simulink model "discrete_kalman_filter"  (R2015b)
settings: Solver=VariableStepAuto  StartTime=0.0  StopTime=10.0  RelTol=1e-3
undefined symbols (not defined in the file or in its folder): KF_A, KF_B, KF_C, KF_D, KF_h, KF_P0, KF_Q, KF_R, KF_x0
settings Model: Creator=mgreiff  LastModifiedBy=mgreiff

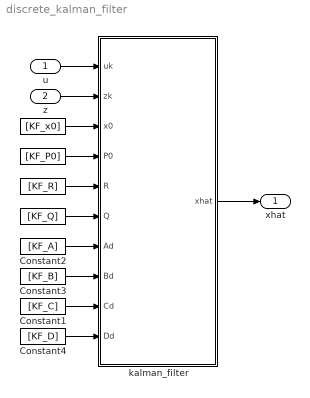
== system discrete_kalman_filter ==
  u : Inport  PortDimensions=4
  z : Inport  Port=2  PortDimensions=9
  " " : Constant  Value=[KF_P0]
  "  " : Constant  Value=[KF_R]
  "   " : Constant  Value=[KF_Q]
  "          " : Constant  Value=[KF_x0]
  Constant1 : Constant  Value=[KF_C]
  Constant2 : Constant  Value=[KF_A]
  Constant3 : Constant  Value=[KF_B]
  Constant4 : Constant  Value=[KF_D]
  kalman_filter : MATLAB Function  TreatAsAtomicUnit=on  SystemSampleTime=KF_h
  xhat : Outport  PortDimensions=12
  wires:
  u/1 -> kalman_filter/1(uk)
  z/1 -> kalman_filter/2(zk)
  " "/1 -> kalman_filter/4(P0)
  "  "/1 -> kalman_filter/5(R)
  "   "/1 -> kalman_filter/6(Q)
  kalman_filter/1(xhat) -> xhat/1
  Constant1/1 -> kalman_filter/9(Cd)
  "          "/1 -> kalman_filter/3(x0)
  Constant4/1 -> kalman_filter/10(Dd)
  Constant3/1 -> kalman_filter/8(Bd)
  Constant2/1 -> kalman_filter/7(Ad)

== matlab function discrete_kalman_filter/kalman_filter ==
  data: uk input; zk input; xhat output; x0 input; P0 input; R input; Q input; Ad input; Bd input; Cd input; Dd input
function xhat  = fcn(uk, zk, x0, P0, R, Q, Ad, Bd, Cd, Dd)
%#codegen
% xkm1  = [x,             uk = [omega_1,         zk = Cd*xkm1
%          y,                   omega_2,      
%          z,                   omega_3,       
%          dotx,                omega_4] 
%          doty,                                  
%          dotz,                                   
%          phi,
%          theta,
%          dotphi,
%          dottheta]

persistent P
persistent xm1

if isempty(P)
    P = P0;
    xm1 = x0;
end

% Predictor step
xf = Ad * xm1 + Bd * uk;
Pf = Ad * P * Ad' + Q;

% Corrector step
K =  Pf * Cd' / (Cd * Pf * Cd'+ R);
xhat = xf + K * (zk - Cd * xf);
P = (eye(12) - K * Cd) * Pf;
xm1 = xhat;
